simulink model "MotorTorqueControlTest_working_5_8_2022_ADC_FILT_Mo"  (R2024b)
settings: Solver=FixedStepAuto  StartTime=0.0  StopTime=inf  FixedStep=0.001  RelTol=1e-3  EnableMultiTasking=on
undefined symbols (not defined in the file): mu_X, mu_y, sigma_X, sigma_y
libraries: slrealtimeethercatlib x35, slrealtimeiplib x6, slrealtimeutilitieslib x5, simulink_extras x5, slrealtimeloglib x3, slpidlib x1, simulink x1
(part 4 of 4)

== matlab function MotorTorqueControlTest_working_5_8_2022_ADC_FILT_Mo/Subsystem1/Get Event/get_event ==
  data: minval_old input; maxval_old input; period_old input; last_event_old input; told input; signal_old input; signal input; minval output; tnew input; fall input; mintime input; time_to_hold input; maxval output; period output; last_event output; lev input; newval output; stance_flag output
function [minval, maxval,period,last_event,newval, stance_flag] = get_event(minval_old,maxval_old,period_old,last_event_old,told,signal_old,signal,tnew,fall,mintime,time_to_hold,lev)%(signal,time_stamp,time_to_hold,minval_old,maxval_old)
if (signal-minval_old)/(maxval_old-minval_old) < lev * 1.3
    stance_flag = 1;
else
    stance_flag = 0;
end 

if tnew<=time_to_hold
    minval=min([signal minval_old]);
    maxval=max([signal maxval_old]);
    last_event=last_event_old;
    period=period_old;
    newval = 0;
else
    minval=minval_old;
    maxval=maxval_old;
    %check for new rise
    oldval=(signal_old-minval)/(maxval-minval);
    newval=(signal-minval)/(maxval-minval);
    d=(-1)^fall;
    if (d*newval>d*lev)-(d*oldval>d*lev)==1
        % new rise/fall detected
        time=told+(tnew-told)*(lev-oldval)/((newval-oldval));
        % avoid fake readings
        if (last_event_old==0)
            last_event=time;
            period=period_old;
        elseif ((last_event_old~=0)&&((time-last_event_old)>mintime))
            period=time-last_event_old;
            last_event=time;
        else
            last_event=last_event_old;
            period=period_old;
        end
    else
        last_event=last_event_old;
        period=period_old;
    end
end
end

== matlab function MotorTorqueControlTest_working_5_8_2022_ADC_FILT_Mo/Subsystem1/HIGH LEVEL CONTROL (200 Hz)1/Get Event/get_event ==
  data: minval_old input; maxval_old input; period_old input; last_event_old input; told input; signal_old input; signal input; minval output; tnew input; fall input; mintime input; time_to_hold input; maxval output; period output; last_event output; lev input; newval output
function [minval, maxval,period,last_event,newval] = get_event(minval_old,maxval_old,period_old,last_event_old,told,signal_old,signal,tnew,fall,mintime,time_to_hold,lev)%(signal,time_stamp,time_to_hold,minval_old,maxval_old)
if tnew<=time_to_hold
    minval=min([signal minval_old]);
    maxval=max([signal maxval_old]);
    last_event=last_event_old;
    period=period_old;
    newval = 0;
else
    minval=minval_old;
    maxval=maxval_old;
    %check for new rise
    oldval=(signal_old-minval)/(maxval-minval);
    newval=(signal-minval)/(maxval-minval);
    d=(-1)^fall;
    if (d*newval>d*lev)-(d*oldval>d*lev)==1
        % new rise/fall detected
        time=told+(tnew-told)*(lev-oldval)/((newval-oldval));
        % avoid fake readings
        if (last_event_old==0)
            last_event=time;
            period=period_old;
        elseif ((last_event_old~=0)&&((time-last_event_old)>mintime))
            period=time-last_event_old;
            last_event=time;
        else
            last_event=last_event_old;
            period=period_old;
        end
    else
        last_event=last_event_old;
        period=period_old;
    end
end
end

== matlab function MotorTorqueControlTest_working_5_8_2022_ADC_FILT_Mo/Subsystem1/HIGH LEVEL CONTROL (200 Hz)1/Get Event1/get_event ==
  data: minval_old input; maxval_old input; period_old input; last_event_old input; told input; signal_old input; signal input; minval output; tnew input; fall input; mintime input; time_to_hold input; maxval output; period output; last_event output; lev input
function [minval, maxval,period,last_event] = get_event(minval_old,maxval_old,period_old,last_event_old,told,signal_old,signal,tnew,fall,mintime,time_to_hold,lev)%(signal,time_stamp,time_to_hold,minval_old,maxval_old)
if tnew<=time_to_hold
    minval=min([signal minval_old]);
    maxval=max([signal maxval_old]);
    last_event=last_event_old;
    period=period_old;
else
    minval=minval_old;
    maxval=maxval_old;
    %check for new rise
    oldval=(signal_old-minval)/(maxval-minval);
    newval=(signal-minval)/(maxval-minval);
    d=(-1)^fall;
    if (d*newval<d*lev)-(d*oldval<d*lev)==1
        % new rise/fall detected
        time=told+(tnew-told)*(lev-oldval)/((newval-oldval));
        % avoid fake readings
        if (last_event_old==0)
            last_event=time;
            period=period_old;
        elseif ((last_event_old~=0)&&((time-last_event_old)>mintime))
            period=time-last_event_old;
            last_event=time;
        else
            last_event=last_event_old;
            period=period_old;
        end
    else
        last_event=last_event_old;
        period=period_old;
    end
end
end

== matlab function MotorTorqueControlTest_working_5_8_2022_ADC_FILT_Mo/Triggered Subsystem6/MATLAB Function ==
  data: sig_in input; newbuf output; prev_buf input; N input; prev_updated_idx input; last_updated_idx output
function [newbuf,last_updated_idx]=circ_buffer(sig_in,prev_buf,N,prev_updated_idx)
    newbuf=prev_buf;
    last_updated_idx=next_idx(prev_updated_idx,N);
    newbuf(last_updated_idx)=sig_in;
end

function out=next_idx(t,N)
out=mod(t,N)+1;
end

== matlab function MotorTorqueControlTest_working_5_8_2022_ADC_FILT_Mo/Subsystem1/HIGH LEVEL CONTROL (200 Hz)1/Get Event2/get_event ==
  data: minval_old input; maxval_old input; period_old input; last_event_old input; told input; signal_old input; signal input; minval output; tnew input; fall input; mintime input; time_to_hold input; maxval output; period output; last_event output; lev input
function [minval, maxval,period,last_event] = get_event(minval_old,maxval_old,period_old,last_event_old,told,signal_old,signal,tnew,fall,mintime,time_to_hold,lev)%(signal,time_stamp,time_to_hold,minval_old,maxval_old)
if tnew<=time_to_hold
    minval=min([signal minval_old]);
    maxval=max([signal maxval_old]);
    last_event=last_event_old;
    period=period_old;
else
    minval=minval_old;
    maxval=maxval_old;
    %check for new rise
    oldval=(signal_old-minval)/(maxval-minval);
    newval=(signal-minval)/(maxval-minval);
    d=(-1)^fall;
    if (d*newval<d*lev)-(d*oldval<d*lev)==1
        % new rise/fall detected
        time=told+(tnew-told)*(lev-oldval)/((newval-oldval));
        % avoid fake readings
        if (last_event_old==0)
            last_event=time;
            period=period_old;
        elseif ((last_event_old~=0)&&((time-last_event_old)>mintime))
            period=time-last_event_old;
            last_event=time;
        else
            last_event=last_event_old;
            period=period_old;
        end
    else
        last_event=last_event_old;
        period=period_old;
    end
end
end

== matlab function MotorTorqueControlTest_working_5_8_2022_ADC_FILT_Mo/Subsystem1/HIGH LEVEL CONTROL (200 Hz)1/HIP_assistive_controller/assistance torque calculation/Embedded MATLAB Function ==
  data: T input; Tout output; gain_pos input; gain_neg input
function Tout = fcn(T, gain_pos, gain_neg)
%#eml
% Tout = T;
% Tout(T>0) = T(T>0) *gain_pos;
% Tout(T<0) = T(T<0) *gain_neg;

if T >0
    Tout = T * gain_pos;
else
    Tout = T * gain_neg;
end

== matlab function MotorTorqueControlTest_working_5_8_2022_ADC_FILT_Mo/Subsystem1/HIGH LEVEL CONTROL (200 Hz)1/HIP_assistive_controller/assistance torque calculation/Embedded MATLAB Function1 ==
  data: T input; Tout output; gain_pos input; gain_neg input
function Tout = fcn(T, gain_pos, gain_neg)
%#eml
% Tout = T;
% Tout(T>0) = T(T>0) *gain_pos;
% Tout(T<0) = T(T<0) *gain_neg;

if T >0
    Tout = T * gain_pos;
else
    Tout = T * gain_neg;
end

== matlab function MotorTorqueControlTest_working_5_8_2022_ADC_FILT_Mo/Subsystem1/HIGH LEVEL CONTROL (200 Hz)1/non-linear AFO/non-linear adaptive oscillator/adaptive oscillator/Embedded MATLAB Function ==
  data: meas_pos input; parameters input; coupling input; POstate_out output; POstate_in input; enable input
function POstate_out  = adaptive_osc(meas_pos,parameters,coupling,POstate_in, enable)
if ~enable
    POstate_out = POstate_in;
return
end
% This function implements a discretized version of the simple adaptive oscillator
% for periodic profiles

% inputs: - meas_pos is the measured position
%         - POstate_in is the current state of the main adaptive oscillator
%         - parameters is the parameters vector
%         - coupling is the coupling parameter
%               0 no coupling - 1 hip coupling - 2 knee coupling - 3 hip and knee coupling -
%               4 left and right coupling - 5 all to all coupling
% outputs: - POstate_out is the updated state of the main adaptive oscillator

%% PARAMETERS
eps = parameters(1);    % coupling constant (speed of phase synchronization to F(t))
nu = parameters(2);     % integrator gain
stime = parameters(3);  % sampling time [s]
nbr_osc = 6;           % number of oscillators

%%%%%%%%%%%%%%%%%%%%%%%%%%%%%%%%%%%%%%%%%%%%%%%%%%%%%%%%%%%%%%%%%%%%%%%%%%%
%  ??? perchè ci sono 6 oscillatori ? corrispondono alle condizioni di
%  couplings? che senso ha?
%%%%%%%%%%%%%%%%%%%%%%%%%%%%%%%%%%%%%%%%%%%%%%%%%%%%%%%%%%%%%%%%%%%%%%%%%%%

%% PHASE OSCILLATOR STATE
offset  = POstate_in(1,:);              % alpha0(t)
omega   = POstate_in(2,:);              % frequency of the oscillator
phi     = POstate_in(3:2+nbr_osc,:);    % phase of the oscillator 
ampl    = POstate_in(3+nbr_osc:end,:);  % amplitude of the oscillator (alpha1(t))

%% ITERATION LOOP

%%%%%%%%%%%%%%%%%%%%%%%%%%%%%%%%%%%%%%%%%%%%%%%%%%%%%%%%%%%%%%%%%%%%%%%%%%%
% DEFINIGN TECHING SIGNAL
%%%%%%%%%%%%%%%%%%%%%%%%%%%%%%%%%%%%%%%%%%%%%%%%%%%%%%%%%%%%%%%%%%%%%%%%%%%
% teaching signals: F(t) = theta_measured - theta_estimated
% theta_measured = meas_pos
% theta estimated = offset + ampl * sin(phi(t))
teach_signal = meas_pos - offset - sum(ampl.*sin(phi),1);   


%%%%%%%%%%%%%%%%%%%%%%%%%%%%%%%%%%%%%%%%%%%%%%%%%%%%%%%%%%%%%%%%%%%%%%%%%%%
%  UPDATE OSCILLATOR PARAMETERS
%%%%%%%%%%%%%%%%%%%%%%%%%%%%%%%%%%%%%%%%%%%%%%%%%%%%%%%%%%%%%%%%%%%%%%%%%%%
% update phi to the current iteration:
% phi(t+1) = phi(t) + stima * (omega(t) + eps * teach_signal(t) * cos(phi(t)))
new_phi = mod( phi + stime*(repmat((1:nbr_osc)',1,4).*repmat(omega,nbr_osc,1) + eps*repmat(teach_signal,nbr_osc,1).*cos(phi)) , 2*pi);
% nota: il modo viene preso perchè phi è una fase percui deve essere
% compresa quindi per definizione tra 0 e 2*pi 

% update omega to the current iteration:
% omega(t+1) = omega(t) * stime * ( eps * teach_signal(t) * cos(phi(t)) )
new_omega = omega + stime*(eps*teach_signal.*cos(phi(1,:)));

% update the amplitide to the current iteration:
% ampl(t+1) = ampl(t) + stime * (nu * theach_signal(t) * sin (phi(t)) )
new_ampl = ampl + stime*(nu*repmat(teach_signal,nbr_osc,1).*sin(phi));

% update the offset to the current iteration:
% offset(t+1) = offset(t) + stime * ( nu * teachsignal(t) )
new_offset = offset + stime*(nu*teach_signal);

%%%%%%%%%%%%%%%%%%%%%%%%%%%%%%%%%%%%%%%%%%%%%%%%%%%%%%%%%%%%%%%%%%%%%%%%%%%
% COUPLING BETWEEN DIFFERENT JOINTS
%%%%%%%%%%%%%%%%%%%%%%%%%%%%%%%%%%%%%%%%%%%%%%%%%%%%%%%%%%%%%%%%%%%%%%%%%%%

% ATTENZIONE: qua non mi torna che si faccia la media anche su ampiezza ed
% offset dell'oscillatore infatti secondo me si introduce un errore nella
% stima (per il fatto che anca e ginocchio possono avere ampiezze diverse)
% che riduce la capacità dell'AFO di trackare il segnale

switch coupling
    case 1,
        new_omega(:,1:2) = repmat(mean(new_omega(:,1:2),2),1,2);
        new_ampl(:,1:2) = repmat(mean(new_ampl(:,1:2),2),1,2);
        new_offset(:,1:2) = repmat(mean(new_offset(:,1:2),2),1,2);
    case 2,        
        new_omega(:,3:4) = repmat(mean(new_omega(:,3:4),2),1,2);
        new_ampl(:,3:4) = repmat(mean(new_ampl(:,3:4),2),1,2);
        new_offset(:,3:4) = repmat(mean(new_offset(:,3:4),2),1,2);
    case 3,
        new_omega(:,1:2) = repmat(mean(new_omega(:,1:2),2),1,2);
        new_ampl(:,1:2) = repmat(mean(new_ampl(:,1:2),2),1,2);
        new_offset(:,1:2) = repmat(mean(new_offset(:,1:2),2),1,2);
        new_omega(:,3:4) = repmat(mean(new_omega(:,3:4),2),1,2);
        new_ampl(:,3:4) = repmat(mean(new_ampl(:,3:4),2),1,2);
        new_offset(:,3:4) = repmat(mean(new_offset(:,3:4),2),1,2);
    case 4,
        new_omega(:,[1 3]) = repmat(mean(new_omega(:,[1 3]),2),1,2);
        new_omega(:,[2 4]) = repmat(mean(new_omega(:,[2 4]),2),1,2);
    case 5,
        new_omega = repmat(mean(new_omega,2),1,4);
        new_ampl(:,1:2) = repmat(mean(new_ampl(:,1:2),2),1,2);
        new_offset(:,1:2) = repmat(mean(new_offset(:,1:2),2),1,2);
        new_ampl(:,3:4) = repmat(mean(new_ampl(:,3:4),2),1,2);
        new_offset(:,3:4) = repmat(mean(new_offset(:,3:4),2),1,2);
end

% % riga modificata da TL l' 8/8/2011
% Omega RESET:
% evita che l'scillatore sia attratto dalla frequenza 0
% se scende sotto 0.1 Hz viene riprotato a 0.8 Hz in modo secco
for i = 1:size(new_omega,1)
    for j = 1:size(new_omega,2)
        if new_omega(i,j)< (0.1*2*pi)
            new_omega(i,j) = 0.8*2*pi;
        end
    end
end
% NOTA: per come era scritta prima prevedeva di utilizzare vettori dalla
% lunghezza variabile
%
% % riga senza find 
% new_omega(new_omega<0.1*2*pi) = 0.8*2*pi;


% riga originale: 
% new_omega(find(new_omega<0.1*2*pi)) = 0.8*2*pi;

POstate_out = [new_offset; new_omega; new_phi; new_ampl];

== matlab function MotorTorqueControlTest_working_5_8_2022_ADC_FILT_Mo/Subsystem1/HIGH LEVEL CONTROL (200 Hz)1/non-linear AFO/non-linear adaptive oscillator/non linear filter/Embedded MATLAB Function ==
  data: meas_pos input; est_pos output; phi input; delta_phase input; lambda input; c_kernel input; h input; coupling input; P_in input; w_in input; delta_pos output; P_out output; w_out output
function [est_pos,delta_pos,P_out,w_out] = ...
    nonlin_filter(meas_pos,phi,delta_phase,lambda,c_kernel,h,coupling,P_in,w_in)

% This function implements a discretized version of the adaptive non-linear filter of the adaptive oscillator
% for non-sinusoidal profiles

% inputs: - meas_pos is the measured position
%         - phi are the current phase of the adaptive oscillator
%         - delta_phase is the phase lead/lag to estimate the position
%         - lambda is the forgetting factor of the recursive least-square to determine weigth_i
%         - c_kernel is a vector with the centers of the gaussian-like functions of the kernel
%         - h is a constant that specifies the width of the gaussian-like functions of the kernel 
%         - parameters is the vector of parameters
%         - coupling is the coupling condition:
%               0 no coupling - 1 hip coupling - 2 knee coupling - 3 hip and knee coupling
%         - P_in and w_in are the state vectors of the local filter
% 
% 
% outputs: - est_pos is the real-time estimated (filtered) output
%          - delta_pos is the lead/lag estimated (filtered) output
%          - P_out and w_out are the state vectors of the local filter


%%%%%%%%%%%%%%%%%%%%%%%%%%%%%%%%%%%%%%%%%%%%%%%%%%%%%%%%%%%%%%%%%%%%%%%%%%%
% To estimate the envelope of the non-sinusoidal profile a pool of adaptive
% oscillators is coupled to a kernel-based non-linear filter.
% 
% The following supervised learning problem is formulated:
% 
% theta_estimate = sommatoria( psi_i(phi(t)) *weight_i) 
%                     / sommatotia( psi_i(phi(t)) );
% 
% where psi_i(phi(t)) = exp( h *( cos( phi(t)-c_i ) - 1 ) )
% h = constant parameter that determines the width of the gaussian curve
% c_i = constant parameters that determine the position of the centers
% 
% Using incremental regression an on-line version of the learing problem
% can be formulated. (using recursive least-squares with forgetting factor
% lambda to deternmine the weigths (weigth_i) )
% Specifically:
% weigth_i(t+1) = weigth_i(t) + psi_i(phi(t)) * P_i(t+1) * (theta_meas(t) -weigth_i(t))
% 
% where P_i(t+1) = ( P_i(t) - ( P_i(t)^2 / ( (lambda /psi_i(phi(t)) + P_i(t) ) ) /lambda; 

% NOTE that P_i is the inverse of the covariance matrix
% lambda = forgetting factor (lambda<1 gives more weigth to recent data)
%%%%%%%%%%%%%%%%%%%%%%%%%%%%%%%%%%%%%%%%%%%%%%%%%%%%%%%%%%%%%%%%%%%%%%%%%%%


% ITERATION LOOP

%%%%%%%%%%%%%%%%%%%%%%%%%%%%%%%%%%%%%%%%%%%%%%%%%%%%%%%%%%%%%%%%%%%%%%%%%%%
% psi is calculated for all the gaussina-like functions (all i)
psi = exp(h*(cos(repmat(phi,length(c_kernel),1)-repmat(c_kernel,1,4))-1));


%%%%%%%%%%%%%%%%%%%%%%%%%%%%%%%%%%%%%%%%%%%%%%%%%%%%%%%%%%%%%%%%%%%%%%%%%%%
% P_out = inverse covariance matrix for t+1
P_out = 1/lambda*(P_in-P_in.^2./(lambda./psi+P_in));


%%%%%%%%%%%%%%%%%%%%%%%%%%%%%%%%%%%%%%%%%%%%%%%%%%%%%%%%%%%%%%%%%%%%%%%%%%%
% w = weigths (all i) of the kernel functions
% allocate memory
w_out = NaN(length(c_kernel),4);

w_out(:,1) = w_in(:,1) + psi(:,1).*P_out(:,1).*(meas_pos(1)-w_in(:,1));

if coupling == 1 || coupling == 3,
    w_out(:,1) = w_out(:,1) + psi(:,2).*P_out(:,2).*(meas_pos(2)-w_in(:,2));
    w_out(:,2) = w_out(:,1);
else
    w_out(:,2) = w_in(:,2) + psi(:,2).*P_out(:,2).*(meas_pos(2)-w_in(:,2));
end

w_out(:,3) = w_in(:,3) + psi(:,3).*P_out(:,3).*(meas_pos(3)-w_in(:,3));
if coupling == 2 || coupling == 3,
    w_out(:,3) = w_out(:,3) + psi(:,4).*P_out(:,4).*(meas_pos(4)-w_in(:,4));
    w_out(:,4) = w_out(:,3);
else
    w_out(:,4) = w_in(:,4) + psi(:,4).*P_out(:,4).*(meas_pos(4)-w_in(:,4));
end


%%%%%%%%%%%%%%%%%%%%%%%%%%%%%%%%%%%%%%%%%%%%%%%%%%%%%%%%%%%%%%%%%%%%%%%%%%%
% estimated position
est_pos = sum(psi.*w_out,1)./sum(psi,1);


%%%%%%%%%%%%%%%%%%%%%%%%%%%%%%%%%%%%%%%%%%%%%%%%%%%%%%%%%%%%%%%%%%%%%%%%%%%
% phase lead/lag

% calculate psi value for the phase lead/lag
psi_shift = exp(h*(cos(repmat(phi,length(c_kernel),1)+delta_phase-repmat(c_kernel,1,4))-1));

% calculate the estimated lead/lag position
delta_pos = sum(psi_shift.*w_out,1)./sum(psi_shift,1);

== matlab function MotorTorqueControlTest_working_5_8_2022_ADC_FILT_Mo/Triggered Subsystem6/MATLAB Function2 ==
  data: y output; data input; y_buffer output; y_buffer input; i input; i output
function [y, y_buffer, i] = fcn(data, y_buffer, i)

if abs(data-y_buffer(1))>10 && abs(data-y_buffer(2))>10 && abs(data-y_buffer(3))>10 && abs(data-y_buffer(4))>10 && abs(data-y_buffer(5))>10
    y = y_buffer(rem(i,5)+1); 
    return;
end
y_buffer(rem(i,5)+1) = data;
i = i+1;
y = data;

== matlab function MotorTorqueControlTest_working_5_8_2022_ADC_FILT_Mo/Triggered Subsystem6/MATLAB Function1 ==
  data: sig_in input; newbuf output; prev_buf input; N input; prev_updated_idx input; last_updated_idx output
function [newbuf,last_updated_idx]=circ_buffer(sig_in,prev_buf,N,prev_updated_idx)
    newbuf=prev_buf;
    last_updated_idx=next_idx(prev_updated_idx,N);
    newbuf(last_updated_idx)=sig_in;
end

function out=next_idx(t,N)
out=mod(t,N)+1;
end

== stateflow chart MotorTorqueControlTest_working_5_8_2022_ADC_FILT_Mo/Motor Initliazation ==
  state inits
    entry:
    Controlword = 0;
  note: The first commandword to the motor must be 0!
  state inits1
    entry:
    Controlword = 6;
  state inits3
    entry:
    Controlword = 128;
  note: If the model starts with the motor in Fault stat
      | this block will attempt to clear it
  state inits4
    entry:
    Controlword = 7;
  state inits2
    entry:
    Controlword = 15;
  (default) -> inits
  inits3 -> inits : [Stateword == 1632]
  inits -> (junction 12) [order 2]
  inits2 -> inits [order 2] : [Stateword == 999| Stateword == 64]
  inits1 -> inits [order 3] : [Stateword == 999 | Stateword == 64 ]
  inits -> inits1 [order 1] : [Stateword == 1632]
  inits1 -> (junction 12) [order 2]
  (junction 12) -> inits3 : [Stateword == 1576 |Stateword == 8]
  inits2 -> (junction 12) [order 1]
  inits1 -> inits4 [order 1] : [Stateword == 1569]
  inits4 -> inits2 : [Stateword == 1571]
  data: Stateword input; Controlword output
